simulink model "Day30"  (R2024b)
settings: Solver=VariableStepAuto  StartTime=0.0  StopTime=10.0  RelTol=1e-3
settings Model: Creator=jun_mac  LastModifiedBy=jun_mac

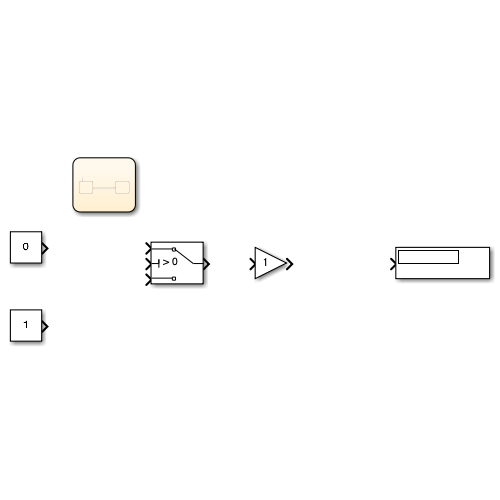
[thumbnail: Simulink's stored preview of the top-level diagram]
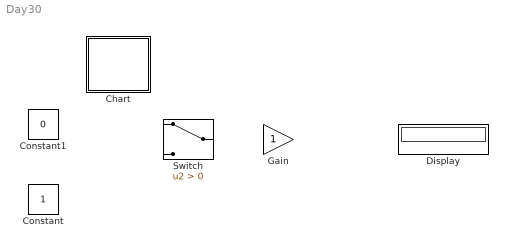
== system Day30 ==
  Chart : Stateflow chart  TreatAsAtomicUnit=on
  Constant : Constant
  Constant1 : Constant  Value=0
  Display : Display
  Gain : Gain
  Switch : Switch  Criteria=u2 > Threshold  SaturateOnIntegerOverflow=off  InputSameDT=off

== stateflow chart Day30/Chart ==
  state LKA_ON
    entry:
    LKA=1;
  state LKA_OFF
    entry:
    LKA=0;
  (default) -> LKA_ON
  LKA_ON -> LKA_OFF : [TurnSignal==1]
  LKA_OFF -> LKA_ON : [TurnSignal==0]
